simulink model "Modelo_dinamico"  (R2024a)
settings: Solver=VariableStepAuto  StartTime=0.0  StopTime=5  MaxStep=0.001  RelTol=1e-3
settings Model: Creator=alfre
settings RTWCC: GPUComputeCapability=3.5

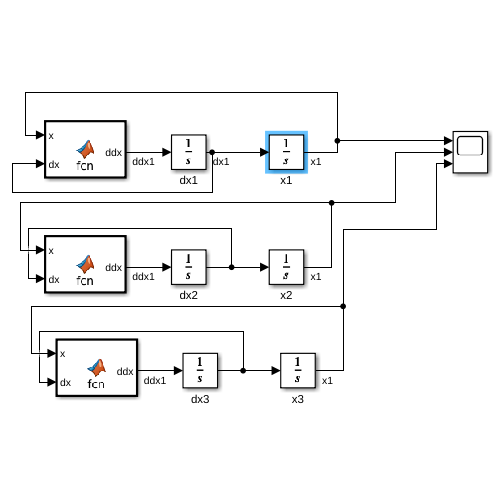
[thumbnail: Simulink's stored preview of the top-level diagram]
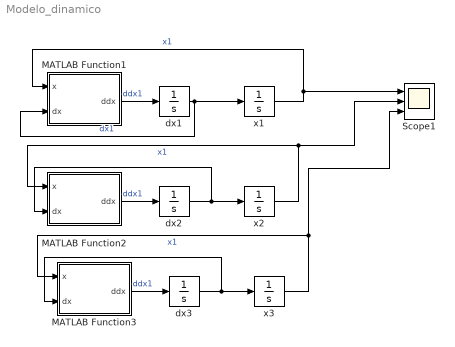
== system Modelo_dinamico ==
  MATLAB Function1 : MATLAB Function  TreatAsAtomicUnit=on
  MATLAB Function2 : MATLAB Function  TreatAsAtomicUnit=on
  MATLAB Function3 : MATLAB Function  TreatAsAtomicUnit=on
  Scope1 : Scope  NumInputPorts=3
  dx1 : Integrator  ContinuousStateAttributes="\"dx\""
  dx2 : Integrator  ContinuousStateAttributes="\"dx\""
  dx3 : Integrator  ContinuousStateAttributes="\"dx\""
  x1 : Integrator  InitialCondition=2*pi  ContinuousStateAttributes="\"dx\""
  x2 : Integrator  InitialCondition=2*pi  ContinuousStateAttributes="\"dx\""
  x3 : Integrator  InitialCondition=2*pi  ContinuousStateAttributes="\"dx\""
  wires:
  MATLAB Function1/1(ddx) -> dx1/1  "ddx1"
  dx1/1 -> MATLAB Function1/2(dx), x1/1  "dx1"
  x1/1 -> MATLAB Function1/1(x), Scope1/1  "x1"
  MATLAB Function2/1(ddx) -> dx2/1  "ddx1"
  dx2/1 -> MATLAB Function2/2(dx), x2/1
  x2/1 -> Scope1/2, MATLAB Function2/1(x)  "x1"
  MATLAB Function3/1(ddx) -> dx3/1  "ddx1"
  x3/1 -> Scope1/3, MATLAB Function3/1(x)  "x1"
  dx3/1 -> MATLAB Function3/2(dx), x3/1

== matlab function Modelo_dinamico/MATLAB Function2 ==
  data: x input; ddx output; dx input
function ddx = fcn(x, dx)
k=0.01;
m = 0.75;
l = 0.36;
g=9.8;
a=l/2;
Tau= 0.5;
J=(4*m*a^2)/3;
ddx= Tau/J- k*dx/J- m*g*a*x/J;

== matlab function Modelo_dinamico/MATLAB Function3 ==
  data: x input; ddx output; dx input
function ddx = fcn(x, dx)
k=0.01;
m = 0.75;
l = 0.36;
g=9.8;
a=l/2;
Tau= 0.5;
J=(4*m*a^2)/3;
ddx= Tau/J- k*dx/J- m*g*a*cos(x)/J;

== matlab function Modelo_dinamico/MATLAB Function1 ==
  data: x input; ddx output; dx input
function ddx = fcn(x, dx)
k=0.01;
m = 0.75;
l = 0.36;
g=9.8;
a=l/2;
Tau= 0.5;
J=(4*m*a^2)/3;
ddx= Tau/J- k*dx/J- m*g*a*sin(x)/J;
